simulink library "csu_pep_piksi_earth_fixed_packet_lib"  (R2014b)
settings: Solver=ode45  StartTime=0.0  StopTime=10.0  RelTol=1e-3
undefined symbols (not defined in the file): gps_delay_counts, gps_rate_to_noise_std
libraries: util_common_lib x6, util_frame_rotation_lib x1, util_info_lib x1
settings Model: Creator=escrane  LastModifiedBy=mstewart

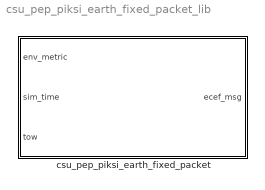
== system csu_pep_piksi_earth_fixed_packet_lib ==
  csu_pep_piksi_earth_fixed_packet : Subsystem

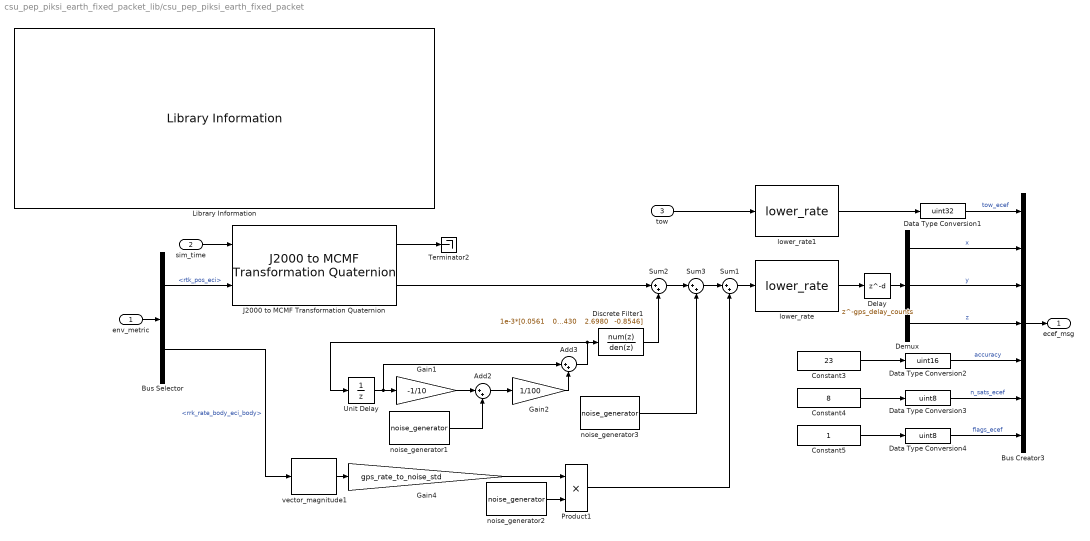
== system csu_pep_piksi_earth_fixed_packet_lib/csu_pep_piksi_earth_fixed_packet ==
  env_metric : Inport
  sim_time : Inport  Port=2
  tow : Inport  Port=3
  Add2 : Sum  Inputs=|++
  Add3 : Sum  Inputs=|++
  Bus Creator3 : BusCreator  Inputs=7
  Bus Selector : BusSelector  OutputSignals=lander_state_bus.rtk_pos_eci,lander_state_bus.rrk_rate_body_eci_body
  Constant3 : Constant  Value=23  OutDataTypeStr=double
  Constant4 : Constant  Value=8  OutDataTypeStr=double
  Constant5 : Constant  OutDataTypeStr=double
  Data Type Conversion1 : DataTypeConversion  OutDataTypeStr=uint32
  Data Type Conversion2 : DataTypeConversion  OutDataTypeStr=uint16
  Data Type Conversion3 : DataTypeConversion  OutDataTypeStr=uint8
  Data Type Conversion4 : DataTypeConversion  OutDataTypeStr=uint8
  Delay : Delay  DelayLength=gps_delay_counts  InitialCondition=0
  Demux : Demux  Outputs=3
  Discrete Filter1 : DiscreteFilter  Numerator="1e-3*[0.0561    0.1682    0.1682    0.0561]"  Denominator="[1.0000   -2.8430    2.6980   -0.8546]"
  Gain1 : Gain  Gain=-1/10
  Gain2 : Gain  Gain=1/100
  Gain4 : Gain  Gain=gps_rate_to_noise_std
  J2000 to MCMF Transformation Quaternion : util_frame_rotation_lib/J2000 to MCMF  Transformation Quaternion  SystemSampleTime=-1
  Library Information : util_info_lib/Library Information  owner='escrane'
  Product1 : Product
  Sum1 : Sum  Inputs=|++
  Sum2 : Sum  Inputs=|++
  Sum3 : Sum  Inputs=|++
  Terminator2 : Terminator
  Unit Delay : UnitDelay  SampleTime=-1
  lower_rate : util_common_lib/lower_rate  counter_max=10  counter_init=0
  lower_rate1 : util_common_lib/lower_rate  counter_max=10  counter_init=0
  noise_generator1 : util_common_lib/noise_generator  std_dev=1  bias=gps_walk_bias_meters  seed=gps_walk_noise_seed_number  on=gps_walk_noise_on  sample_time=sim_time_step_size
  noise_generator2 : util_common_lib/noise_generator  std_dev=1  bias=0  seed=gps_noise_seed_number  on=gps_noise_on  sample_time=sim_time_step_size
  noise_generator3 : util_common_lib/noise_generator  std_dev=5  bias=0  seed=[23 24 25]  on=1  sample_time=sim_time_step_size
  vector_magnitude1 : util_common_lib/vector_magnitude  SystemSampleTime=-1
  ecef_msg : Outport
  wires:
  Bus Creator3/1 -> ecef_msg/1
  Data Type Conversion4/1 -> Bus Creator3/7  "flags_ecef"
  Constant5/1 -> Data Type Conversion4/1
  Data Type Conversion3/1 -> Bus Creator3/6  "n_sats_ecef"
  Constant4/1 -> Data Type Conversion3/1
  Data Type Conversion2/1 -> Bus Creator3/5  "accuracy"
  Constant3/1 -> Data Type Conversion2/1
  Data Type Conversion1/1 -> Bus Creator3/1  "tow_ecef"
  lower_rate1/1 -> Data Type Conversion1/1
  Demux/3 -> Bus Creator3/4  "z"
  Demux/2 -> Bus Creator3/3  "y"
  Demux/1 -> Bus Creator3/2  "x"
  Delay/1 -> Demux/1
  lower_rate/1 -> Delay/1
  Product1/1 -> Sum1/2
  J2000 to MCMF Transformation Quaternion/1 -> Terminator2/1
  sim_time/1 -> J2000 to MCMF Transformation Quaternion/1
  env_metric/1 -> Bus Selector/1
  noise_generator1/1 -> Add2/2
  Gain1/1 -> Add2/1
  Add3/1 -> Unit Delay/1, Discrete Filter1/1
  Unit Delay/1 -> Add3/1, Gain1/1
  Gain2/1 -> Add3/2
  Add2/1 -> Gain2/1
  Bus Selector/1 -> J2000 to MCMF Transformation Quaternion/2  "<rtk_pos_eci>"
  Sum1/1 -> lower_rate/1
  vector_magnitude1/1 -> Gain4/1
  Gain4/1 -> Product1/1
  noise_generator2/1 -> Product1/2
  Bus Selector/2 -> vector_magnitude1/1  "<rrk_rate_body_eci_body>"
  J2000 to MCMF Transformation Quaternion/2 -> Sum2/1
  Discrete Filter1/1 -> Sum2/2
  tow/1 -> lower_rate1/1
  noise_generator3/1 -> Sum3/2
  Sum3/1 -> Sum1/1
  Sum2/1 -> Sum3/1
